simulink model "myproject_task"  (Simulink 3.00)
libraries: mathlib x4, mylibrary x4

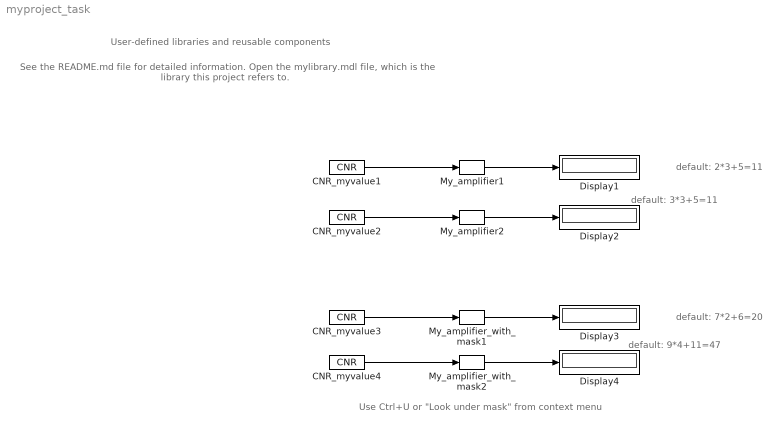
== system myproject_task ==
  note: default: 2*3+5=11
  note: default: 3*3+5=11
  note: default: 7*2+6=20
  note: default: 9*4+11=47
  note: Use Ctrl+U or
      | "Look under mask"
      | from context menu
  note: User-defined libraries and reusable components
  note: See the README.md file for detailed information.
      |
      | Open the mylibrary.mdl file, which is the library this project refers to.
  CNR_myvalue1 : mathlib/CNR  ycn=2
  CNR_myvalue2 : mathlib/CNR  ycn=3
  CNR_myvalue3 : mathlib/CNR  ycn=7
  CNR_myvalue4 : mathlib/CNR  ycn=9
  Display{1..4} (4 alike) : Display
      settings: Format=short
  My_amplifier1 : mylibrary/My_amplifier
      mask Type: REX sequence
  My_amplifier2 : mylibrary/My_amplifier
      mask Type: REX sequence
  My_amplifier_with_mask1 : mylibrary/My_amplifier_with_mask  user_gain=2  user_offset=6
  My_amplifier_with_mask2 : mylibrary/My_amplifier_with_mask  user_gain=4  user_offset=11
  wires:
  CNR_myvalue1/1 -> My_amplifier1/1
  CNR_myvalue2/1 -> My_amplifier2/1
  CNR_myvalue3/1 -> My_amplifier_with_mask1/1
  CNR_myvalue4/1 -> My_amplifier_with_mask2/1
  My_amplifier1/1 -> Display1/1
  My_amplifier2/1 -> Display2/1
  My_amplifier_with_mask1/1 -> Display3/1
  My_amplifier_with_mask2/1 -> Display4/1
